simulink model "project2"  (R2022b)
settings: Solver=VariableStepAuto  StartTime=0.0  StopTime=50  RelTol=1e-3
settings Model: Creator=hayden  LastModifiedBy=hayden

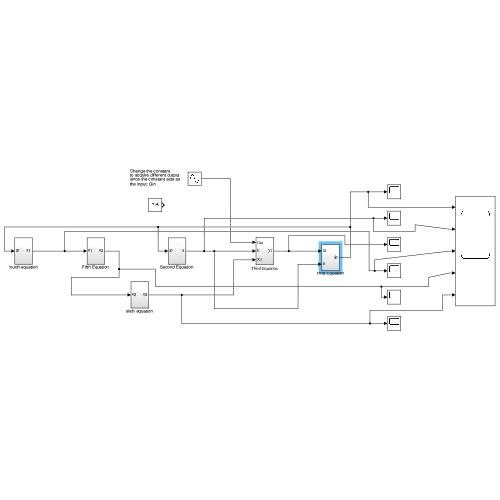
[thumbnail: Simulink's stored preview of the top-level diagram]
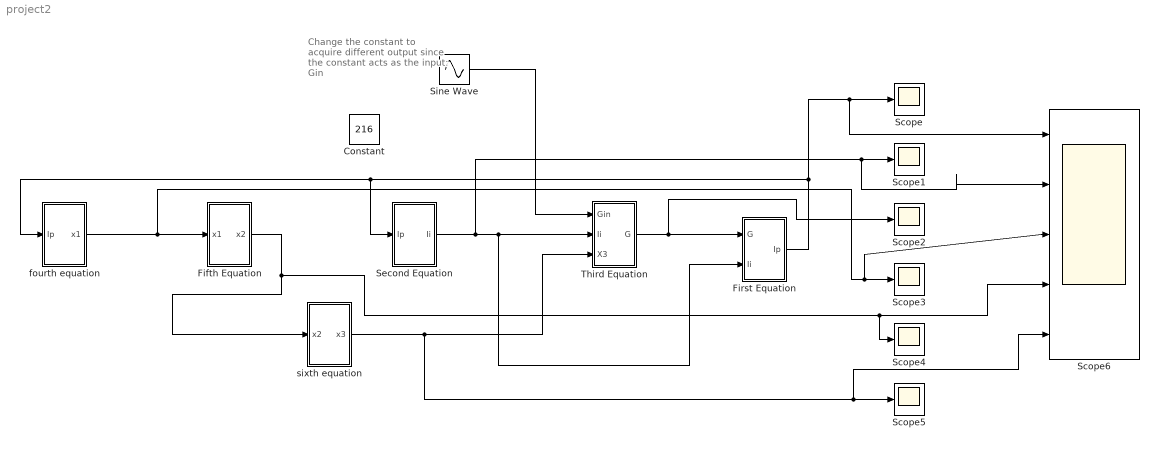
== system project2 ==
  note: Change the constant
      | to acquire different output
      | since the constant acts as
      | the input: Gin
  Constant : Constant  Value=216
  Fifth Equation : Subsystem
  First Equation : Subsystem
  Scope{,1..5} (6 alike) : Scope
  Scope6 : Scope  NumInputPorts=5
  Second Equation : Subsystem
  Sine Wave : Sin  Amplitude=200  SampleTime=0
  Third Equation : Subsystem
  fourth equation : Subsystem
  sixth equation : Subsystem
  wires:
  Third Equation/1(G) -> Scope2/1, First Equation/1(G)
  First Equation/1(Ip) -> Scope6/1, Scope/1, fourth equation/1(Ip), Second Equation/1(Ip)
  Second Equation/1(Ii) -> Scope6/2, Scope1/1, First Equation/2(Ii), Third Equation/2(Ii)
  fourth equation/1(x1) -> Scope6/3, Scope3/1, Fifth Equation/1(x1)
  Fifth Equation/1(x2) -> Scope6/4, Scope4/1, sixth equation/1(x2)
  sixth equation/1(x3) -> Third Equation/3(X3), Scope6/5, Scope5/1
  Sine Wave/1 -> Third Equation/1(Gin)

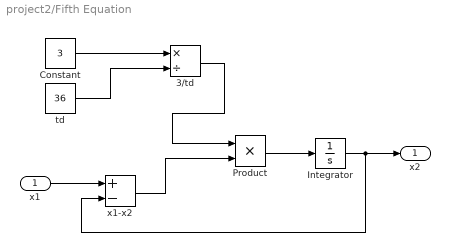
== system project2/Fifth Equation ==
  x1 : Inport
  3/td : Product  Inputs=*/
  Constant : Constant  Value=3
  Integrator : Integrator  InitialCondition=.2
  Product : Product
  td : Constant  Value=36
  x1-x2 : Sum  Inputs=+-
  x2 : Outport
  wires:
  Constant/1 -> 3/td/1
  td/1 -> 3/td/2
  Integrator/1 -> x1-x2/2, x2/1
  x1/1 -> x1-x2/1
  x1-x2/1 -> Product/2
  3/td/1 -> Product/1
  Product/1 -> Integrator/1

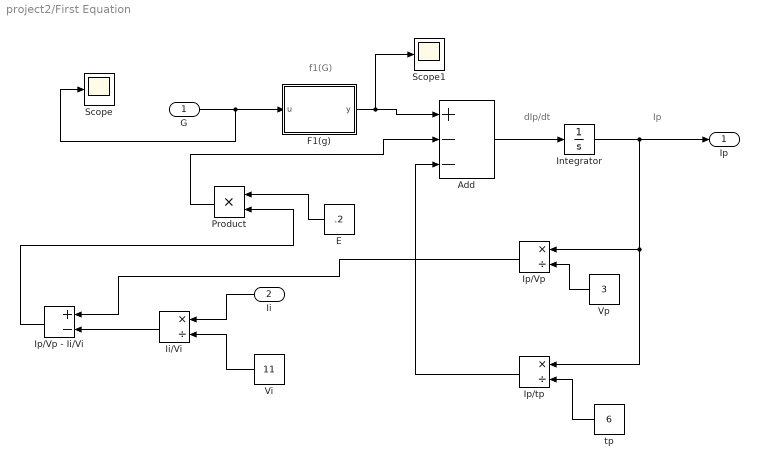
== system project2/First Equation ==
  note: Ip
  note: dIp/dt
  note: f1(G)
  G : Inport
  Ii : Inport  Port=2
  Add : Sum  Inputs=+--
  E : Constant  Value=.2
  F1(g) : MATLAB Function  TreatAsAtomicUnit=on
  Ii/Vi : Product  Inputs=*/
  Integrator : Integrator  InitialCondition=90
  Ip/Vp : Product  Inputs=*/
  Ip/Vp - Ii/Vi : Sum  Inputs=+-
  Ip/tp : Product  Inputs=*/
  Product : Product
  Scope : Scope
  Scope1 : Scope
  Vi : Constant  Value=11
  Vp : Constant  Value=3
  tp : Constant  Value=6
  Ip : Outport
  wires:
  G/1 -> Scope/1, F1(g)/1(u)
  F1(g)/1(y) -> Scope1/1, Add/1
  Add/1 -> Integrator/1
  Integrator/1 -> Ip/tp/1, Ip/Vp/1, Ip/1
  Vp/1 -> Ip/Vp/2
  Ii/1 -> Ii/Vi/1
  Vi/1 -> Ii/Vi/2
  E/1 -> Product/1
  Ii/Vi/1 -> Ip/Vp - Ii/Vi/2
  Ip/Vp/1 -> Ip/Vp - Ii/Vi/1
  Ip/Vp - Ii/Vi/1 -> Product/2
  Product/1 -> Add/2
  tp/1 -> Ip/tp/2
  Ip/tp/1 -> Add/3

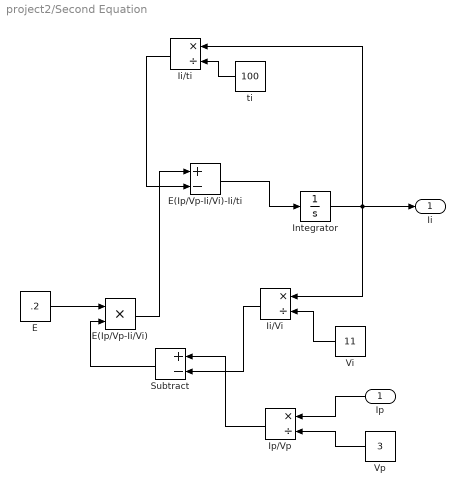
== system project2/Second Equation ==
  Ip : Inport
  E : Constant  Value=.2
  E(Ip/Vp-Ii/Vi) : Product
  E(Ip/Vp-Ii/Vi)-Ii/ti : Sum  Inputs=+-
  Ii/Vi : Product  Inputs=*/
  Ii/ti : Product  Inputs=*/
  Integrator : Integrator  InitialCondition=220
  Ip/Vp : Product  Inputs=*/
  Subtract : Sum  Inputs=+-
  Vi : Constant  Value=11
  Vp : Constant  Value=3
  ti : Constant  Value=100
  Ii : Outport
  wires:
  Integrator/1 -> Ii/ti/1, Ii/Vi/1, Ii/1
  Ip/1 -> Ip/Vp/1
  Vp/1 -> Ip/Vp/2
  Vi/1 -> Ii/Vi/2
  E/1 -> E(Ip/Vp-Ii/Vi)/1
  Subtract/1 -> E(Ip/Vp-Ii/Vi)/2
  ti/1 -> Ii/ti/2
  E(Ip/Vp-Ii/Vi)-Ii/ti/1 -> Integrator/1
  Ii/ti/1 -> E(Ip/Vp-Ii/Vi)-Ii/ti/2
  E(Ip/Vp-Ii/Vi)/1 -> E(Ip/Vp-Ii/Vi)-Ii/ti/1
  Ip/Vp/1 -> Subtract/1
  Ii/Vi/1 -> Subtract/2

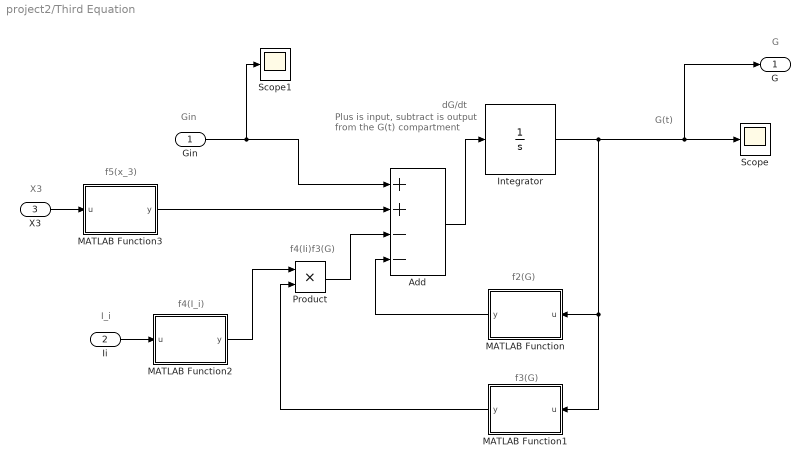
== system project2/Third Equation ==
  note: G
  note: Plus is input, subtract is output
      | from the G(t) compartment
  note: f4(Ii)f3(G)
  note: I_i
  note: X3
  note: Gin
  note: f5(x_3)
  note: f4(I_i)
  note: f3(G)
  note: f2(G)
  note: G(t)
  note: dG/dt
  Gin : Inport
  Ii : Inport  Port=2
  X3 : Inport  Port=3
  Add : Sum  Inputs=++--
  Integrator : Integrator  InitialCondition=12000
  MATLAB Function : MATLAB Function  TreatAsAtomicUnit=on
  MATLAB Function1 : MATLAB Function  TreatAsAtomicUnit=on
  MATLAB Function2 : MATLAB Function  TreatAsAtomicUnit=on
  MATLAB Function3 : MATLAB Function  TreatAsAtomicUnit=on
  Product : Product
  Scope : Scope
  Scope1 : Scope
  G : Outport
  wires:
  Integrator/1 -> MATLAB Function1/1(u), MATLAB Function/1(u), G/1, Scope/1
  Product/1 -> Add/3
  Gin/1 -> Scope1/1, Add/1
  Add/1 -> Integrator/1
  MATLAB Function/1(y) -> Add/4
  MATLAB Function1/1(y) -> Product/2
  Ii/1 -> MATLAB Function2/1(u)
  MATLAB Function2/1(y) -> Product/1
  X3/1 -> MATLAB Function3/1(u)
  MATLAB Function3/1(y) -> Add/2

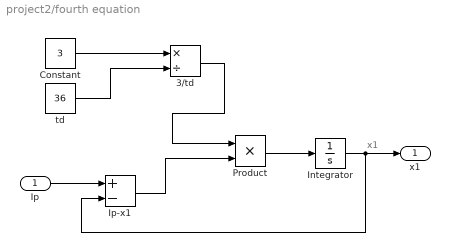
== system project2/fourth equation ==
  note: x1
  Ip : Inport
  3/td : Product  Inputs=*/
  Constant : Constant  Value=3
  Integrator : Integrator  InitialCondition=.1
  Ip-x1 : Sum  Inputs=+-
  Product : Product
  td : Constant  Value=36
  x1 : Outport
  wires:
  Constant/1 -> 3/td/1
  td/1 -> 3/td/2
  Integrator/1 -> Ip-x1/2, x1/1
  Ip/1 -> Ip-x1/1
  Ip-x1/1 -> Product/2
  3/td/1 -> Product/1
  Product/1 -> Integrator/1

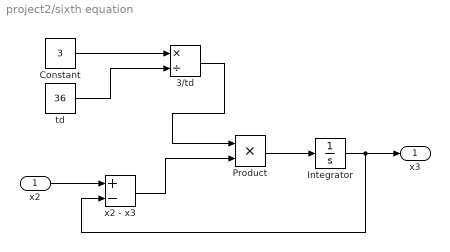
== system project2/sixth equation ==
  x2 : Inport
  3/td : Product  Inputs=*/
  Constant : Constant  Value=3
  Integrator : Integrator  InitialCondition=.1
  Product : Product
  td : Constant  Value=36
  x2 - x3 : Sum  Inputs=+-
  x3 : Outport
  wires:
  Constant/1 -> 3/td/1
  td/1 -> 3/td/2
  Integrator/1 -> x2 - x3/2, x3/1
  x2/1 -> x2 - x3/1
  x2 - x3/1 -> Product/2
  3/td/1 -> Product/1
  Product/1 -> Integrator/1

== matlab function project2/Third Equation/MATLAB Function ==
  data: u input; y output
% f2(g) function
% u = G

function y = fcn(u)
C2 = 144;
Vg = 10;
Ub = 72;

y = Ub*(1-exp(-u/(C2*Vg)));

== matlab function project2/Third Equation/MATLAB Function2 ==
  data: u input; y output
%f4(Ii)
% u = Ii


function y = fcn(u)
Um = 940;
Uo = 40;
Beta = 1.77;
C4 = 80;
Vi = 11;
E = .2;
ti = 100;
%i changed the ti paranthesis
%y = Uo + ((Um - Uo)/(1+exp(-Beta*log(u/C4*(1/Vi+1/E*ti)))));
y = Uo + ((Um - Uo)/(1+exp(-Beta)*(u/C4)*(1/Vi+1/(E*ti))));

== matlab function project2/Third Equation/MATLAB Function3 ==
  data: u input; y output
%f5(x3)
% u = x3

function y = fcn(u)
Rg = 180;
alph = .29;
Vp = 3;
C5 = 26;

y = Rg/(1+exp(alph*(u/Vp - C5)));

== matlab function project2/First Equation/F1(g) ==
  data: u input; y output
%f1(G)
% u = G
function y = fcn(u)
Rm = 210;
C1 = 2000;
Vg = 10;
a1 = 300;

y = Rm/(1+exp((C1 - u/Vg)/a1));

== matlab function project2/Third Equation/MATLAB Function1 ==
  data: u input; y output
%f3(G)
% u = G


function y = fcn(u)
C3 = 1000;
Vg = 10;

y = u/(C3*Vg);
